simulink model "CSTFM_Mclass"  (Simulink 8.5)
settings: Solver=ode1  SolverMode=SingleTasking  StartTime=0.0  StopTime=200  FixedStep=25e-6  RelTol=1e-3
libraries: dspswit3 x1
settings Model: Creator=Administrator  LastModifiedBy=Administrator
settings DataIOCC: SignalLoggingSaveFormat=Dataset  SaveOutput=off  SaveTime=off
settings OptimizationCC: BlockReduction=off  OptimizeBlockIOStorage=off  BufferReuse=off  GlobalBufferReuse=off  ExpressionFolding=off  ExpressionDepthLimit=128  LocalBlockOutputs=off
settings DebuggingCC: UnderspecifiedInitializationDetection=Simplified  MergeDetectMultiDrivingBlocksExec=error  FcnCallInpInsideContextMsg=EnableAllAsError  StateNameClashWarn=none
settings GRTTargetCC: CombineOutputUpdateFcns=on  GRTInterface=off

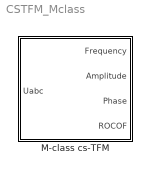
== system CSTFM_Mclass ==
  M-class cs-TFM : Subsystem  SystemSampleTime=2e-4  VariantControl=variant1  mask{nominal_freq=50, Fs=5e3, T=0.1, Fr_50=50}
      mask prompts: nominal_freq "Norminal Frequency"; Fs "Sampling rate (Hz)"; T "Window length (s)"; Fr_50 "Data report rate (frames/s)"
      mask init:
      | %% // PUM initialization//
      | % the file is used to set basic paramters and creat initial matrix  
      | % ** 2018-08-07 YIHUI ZUO
      | 
      | %% basic paramters%
      | %nominal_freq = 50;
      | %T=0.1;
      | TdF=10;
      | % data_rate_50=1; %case: 1(10),2(25),3(50)
      | %Fs=5e3;
      | P=11;
      | 
      | %% creat intial matrix
      | f0 = nominal_freq;
      | 
      | % switch data_rate_50
      | % case 1
      | % Fr_50 = 10;
      | % case 2
      | % Fr_50 = 25;
      | % case 3
      | % Fr_50 = 50;
      | % otherwise
      | % display('Non contemplated data reporting rate')
      | % end
      | 
      | Ts=1/Fs;
      | dF = 1/T;
      | M = round(T*Fs);
      | overlap=4*M/5;
      | kmax = round(f0*T);
      | k = kmax-4:kmax+12;
      | Wk = exp(-1i*2*pi*k./M);
      | NumIters=2;
      | Fr = Fr_50;
      | Tr = 1/Fr;
      | H = M*P;
      | 
      | h_axis = 0:Fs/H:Fs*(H-1)/H; % matrix h_aixs
      | 
      | D = zeros(M,H);%
      | for k = 0:M-1
      |     for h = 0:H-1
      |     esp = k - M*h/H;
      |     esp = esp*(M-1)/M;
      |     a = pi*(k-(h/H)*M);
      |     b = a/M;
      |     if b == pi || b == 0
      |         s = 1;
      |     else
      |         s = sin(a)/(M*sin(b));
      |     end
      |     D(k+1,h+1) = s*exp(-1i*pi*esp);
      |     end
      | end
      | 
      | D_funda=D(2:17,51:61);%
      | D_funda=D_funda'; 
      | inter_index=[12 17 23 28 83 89 94 100];
      | D_inter=D(2:17,inter_index);
      | D_inter=D_inter';
      | f_fund=h_axis(51:61);
      | dft_rec=zeros(11,16);
      | freq=(10:10:160);
      | 
      | for i=1:11
      |     ff0=f_fund(i);
      |     dft_rec(i,:) =(0.5*sinc((freq-ff0)*T)+0.25*sinc((freq-ff0-1/T)*T)+0.25*sinc((freq-ff0+1/T)*T))...
      |     +  (0.5*sinc((-freq+ff0)*T)+0.25*sinc((-freq+ff0-1/T)*T)+0.25*sinc((-freq+ff0+1/T)*T));
      | end
      | 
      | order = 2;
      | M=3*M/5;
      | matrix_f=zeros(M,6,11);%
      | h=1;
      | Nh=M/2;
      | freq=(45:1:55);
      | for index=1:11
      |     omega1=2*pi*freq(index)/Fs;
      |     for i=0:M-1
      |         n = i - Nh;
      |         nc = 0;
      |         facts = factorial(2:-1:0);
      |         e = exp(1j*n*h*omega1);
      |         matrix_f(i+1,nc+1:nc+2*order+2,index) = [(((n*Ts).^(order:-1:0)).*e)./facts, (((n*Ts).^(0:1:order)).*e')./fliplr(facts)];
      |     end
      | end
      | 
      | matrix_har2=zeros(M,6,11); %
      | freq=2*(45:1:55);
      | for index=1:11
      |     omega1=2*pi*freq(index)/Fs;
      |     for i=0:M-1
      |         n = i - Nh;
      |         nc = 0;
      |         facts = factorial(2:-1:0);
      |         e = exp(1j*n*h*omega1);
      |         matrix_har2(i+1,nc+1:nc+2*order+2,index) = [(((n*Ts).^(order:-1:0)).*e)./facts, (((n*Ts).^(0:1:order)).*e')./fliplr(facts)];
      |     end
      | end
      | 
      | matrix_har3=zeros(M,6,11);%
      | freq=3*(45:1:55);
      | for index=1:11
      |     omega1=2*pi*freq(index)/Fs;
      |     for i=0:M-1
      |         n = i - Nh;
      |         nc = 0;
      |         facts = factorial(2:-1:0);
      |         e = exp(1j*n*h*omega1);
      |         matrix_har3(i+1,nc+1:nc+2*order+2,index) = [(((n*Ts).^(order:-1:0)).*e)./facts, (((n*Ts).^(0:1:order)).*e')./fliplr(facts)];
      |     end
      | end
      | 
      | M = round(T*Fs);
      | clear D
      mask TypeOptions Fr_50: 10 | 25 | 50

== system CSTFM_Mclass/M-class cs-TFM ==
  Uabc : Inport
  Buffer : Buffer  N=M  V=overlap  TreatMby1Signals=One channel
  Demux : Demux  Outputs=3
  M-class cs-TFM : Subsystem  TreatAsAtomicUnit=on  SystemSampleTime=Ts*(M-overlap)
  Rate Transition : RateTransition  OutPortSampleTime=2e-4
  Terminator : Terminator
  Terminator1 : Terminator
  msdft Hanning : Subsystem  TreatAsAtomicUnit=on  SystemSampleTime=2e-4
  Frequency : Outport
  Amplitude : Outport  Port=2
  Phase : Outport  Port=3
  ROCOF : Outport  Port=4
  wires:
  Demux/3 -> Terminator1/1
  Demux/2 -> Terminator/1
  Rate Transition/1 -> Buffer/1
  msdft Hanning/1(DFT) -> M-class cs-TFM/2(A)
  M-class cs-TFM/4(RoCoF) -> ROCOF/1
  M-class cs-TFM/3(frequency) -> Frequency/1
  M-class cs-TFM/2(phase_estimated) -> Phase/1
  M-class cs-TFM/1(Amplitude) -> Amplitude/1
  Buffer/1 -> M-class cs-TFM/1(buffer_a)
  Demux/1 -> msdft Hanning/1(signal), Rate Transition/1  "Ua"
  Uabc/1 -> Demux/1

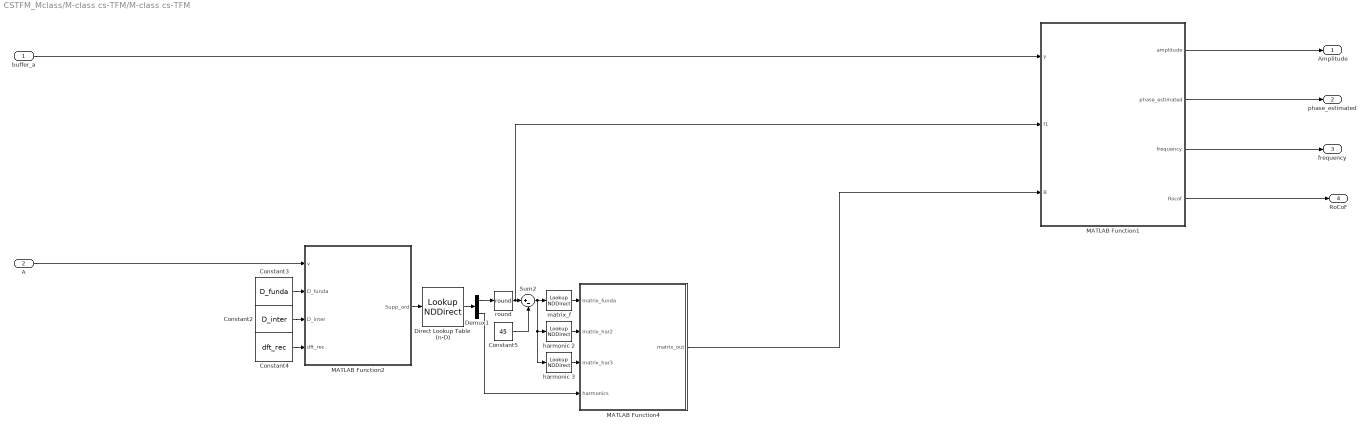
== system CSTFM_Mclass/M-class cs-TFM/M-class cs-TFM ==
  buffer_a : Inport
  A : Inport  Port=2
  Constant2 : Constant  Value=D_inter
  Constant3 : Constant  Value=D_funda
  Constant4 : Constant  Value=dft_rec
  Constant5 : Constant  Value=45
  Demux1 : Demux  Outputs=2
  Direct Lookup Table (n-D) : LookupNDDirect  NumberOfTableDimensions=1  Table=h_axis
  MATLAB Function1 : MATLAB Function  RequirementInfo={} %GIDa_19990d1e_36bc_402c_ae7c_789240e7275e  SystemSampleTime=Ts*(M-overlap)
  MATLAB Function2 : MATLAB Function  SystemSampleTime=Ts*(M-overlap)
  MATLAB Function4 : MATLAB Function  RequirementInfo={} %GIDa_4e17b5a7_f5ca_4ce2_b340_35974142e702  SystemSampleTime=Ts*(M-overlap)
  Sum2 : Sum  Inputs=|+-
  harmonic 2 : LookupNDDirect  NumberOfTableDimensions=3  InputsSelectThisObjectFromTable=2-D Matrix  Table=matrix_har2
  "harmonic 3 " : LookupNDDirect  NumberOfTableDimensions=3  InputsSelectThisObjectFromTable=2-D Matrix  Table=matrix_har3
  matrix_f : LookupNDDirect  NumberOfTableDimensions=3  InputsSelectThisObjectFromTable=2-D Matrix  Table=matrix_f
  round : Rounding  Operator=round
  Amplitude : Outport
  phase_estimated : Outport  Port=2
  frequency : Outport  Port=3
  RoCoF : Outport  Port=4
  wires:
  buffer_a/1 -> MATLAB Function1/1(y)
  round/1 -> Sum2/1, MATLAB Function1/2(f1)
  Constant3/1 -> MATLAB Function2/2(D_funda)
  MATLAB Function2/1(Supp_ord) -> Direct Lookup Table (n-D)/1
  A/1 -> MATLAB Function2/1(v)
  Constant2/1 -> MATLAB Function2/3(D_inter)
  Constant4/1 -> MATLAB Function2/4(dft_rec)
  Direct Lookup Table (n-D)/1 -> Demux1/1
  Demux1/1 -> round/1
  matrix_f/1 -> MATLAB Function4/1(matrix_funda)
  Sum2/1 -> "harmonic 3 "/1, harmonic 2/1, matrix_f/1
  Constant5/1 -> Sum2/2
  harmonic 2/1 -> MATLAB Function4/2(matrix_har2)
  "harmonic 3 "/1 -> MATLAB Function4/3(matrix_har3)
  MATLAB Function4/1(matrix_out) -> MATLAB Function1/3(B)
  Demux1/2 -> MATLAB Function4/4(harmonics)
  MATLAB Function1/1(amplitude) -> Amplitude/1
  MATLAB Function1/2(phase_estimated) -> phase_estimated/1
  MATLAB Function1/3(frequency) -> frequency/1
  MATLAB Function1/4(Rocof) -> RoCoF/1

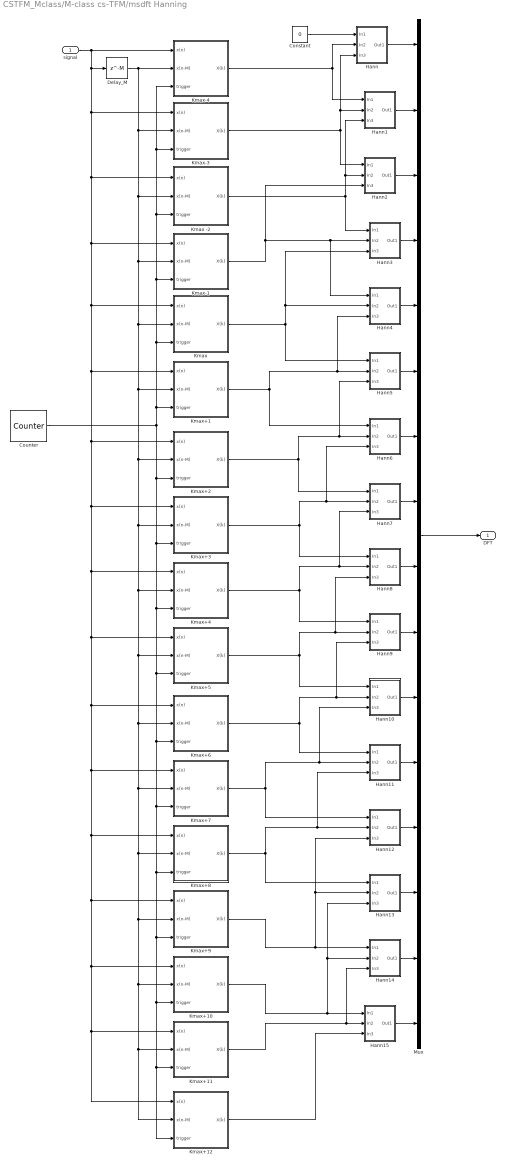
== system CSTFM_Mclass/M-class cs-TFM/msdft Hanning ==
  signal : Inport
  Constant : Constant  Value=0
  Counter : dspswit3/Counter  Direction=Up  CountEvent=Free running  CounterSize=User defined  MaxCount=M-1  InitialCount=1  Output=Hit  HitValue=0  ResetInput=off  SamplesPerFrame=1  Ts=Ts  CntDtype=double  HitDtype=Logical
  Delay_M : Delay  DelayLength=M
  Hann : Subsystem
  Hann1 : Subsystem
  Hann10 : Subsystem
  Hann11 : Subsystem
  Hann12 : Subsystem
  Hann13 : Subsystem
  Hann14 : Subsystem
  Hann15 : Subsystem
  Hann2 : Subsystem
  Hann3 : Subsystem
  Hann4 : Subsystem
  Hann5 : Subsystem
  Hann6 : Subsystem
  Hann7 : Subsystem
  Hann8 : Subsystem
  Hann9 : Subsystem
  Kmax : Subsystem
  Kmax -2 : Subsystem
  Kmax+1 : Subsystem
  Kmax+10 : Subsystem
  Kmax+11 : Subsystem
  Kmax+12 : Subsystem
  Kmax+2 : Subsystem
  Kmax+3 : Subsystem
  Kmax+4 : Subsystem
  Kmax+5 : Subsystem
  Kmax+6 : Subsystem
  Kmax+7 : Subsystem
  Kmax+8 : Subsystem
  Kmax+9 : Subsystem
  Kmax-1 : Subsystem
  Kmax-3 : Subsystem
  Kmax-4 : Subsystem
  Mux : Mux  Inputs=16
  DFT : Outport
  wires:
  Counter/1 -> Kmax+3/3(trigger), Kmax+12/3(trigger), Kmax+11/3(trigger), Kmax+10/3(trigger), Kmax+9/3(trigger), Kmax+8/3(trigger), Kmax+7/3(trigger), Kmax+6/3(trigger), Kmax+5/3(trigger), Kmax+4/3(trigger), Kmax+2/3(trigger), Kmax/3(trigger), Kmax-1/3(trigger), Kmax-3/3(trigger), Kmax-4/3(trigger), Kmax -2/3(trigger), Kmax+1/3(trigger)
  Kmax-4/1(X(k)) -> Hann/2(In2), Hann1/1(In1)
  Kmax-3/1(X(k)) -> Hann2/1(In1), Hann1/2(In2), Hann/3(In3)
  Kmax -2/1(X(k)) -> Hann3/1(In1), Hann2/2(In2), Hann1/3(In3)
  Kmax-1/1(X(k)) -> Hann2/3(In3), Hann4/1(In1), Hann3/2(In2)
  Kmax/1(X(k)) -> Hann4/2(In2), Hann3/3(In3), Hann5/1(In1)
  Kmax+2/1(X(k)) -> Hann7/1(In1), Hann5/3(In3), Hann6/2(In2)
  Kmax+4/1(X(k)) -> Hann9/1(In1), Hann7/3(In3), Hann8/2(In2)
  Kmax+11/1(X(k)) -> Hann14/3(In3), Hann15/2(In2)
  Kmax+10/1(X(k)) -> Hann13/3(In3), Hann14/2(In2), Hann15/1(In1)
  Kmax+9/1(X(k)) -> Hann12/3(In3), Hann13/2(In2), Hann14/1(In1)
  Kmax+8/1(X(k)) -> Hann13/1(In1), Hann11/3(In3), Hann12/2(In2)
  Kmax+7/1(X(k)) -> Hann12/1(In1), Hann10/3(In3), Hann11/2(In2)
  Mux/1 -> DFT/1
  signal/1 -> Kmax+12/1(x(n)), Kmax+11/1(x(n)), Kmax+10/1(x(n)), Kmax+9/1(x(n)), Kmax+8/1(x(n)), Kmax+7/1(x(n)), Kmax+6/1(x(n)), Kmax+5/1(x(n)), Kmax+4/1(x(n)), Kmax+3/1(x(n)), Kmax+2/1(x(n)), Kmax+1/1(x(n)), Kmax/1(x(n)), Kmax-1/1(x(n)), Kmax -2/1(x(n)), Kmax-3/1(x(n)), Delay_M/1, Kmax-4/1(x(n))
  Delay_M/1 -> Kmax+3/2(x(n-M)), Kmax+12/2(x(n-M)), Kmax+11/2(x(n-M)), Kmax+10/2(x(n-M)), Kmax+9/2(x(n-M)), Kmax+8/2(x(n-M)), Kmax+7/2(x(n-M)), Kmax+6/2(x(n-M)), Kmax+5/2(x(n-M)), Kmax+4/2(x(n-M)), Kmax+2/2(x(n-M)), Kmax+1/2(x(n-M)), Kmax/2(x(n-M)), Kmax-1/2(x(n-M)), Kmax -2/2(x(n-M)), Kmax-3/2(x(n-M)), Kmax-4/2(x(n-M))
  Hann/1(Out1) -> Mux/1
  Constant/1 -> Hann/1(In1)
  Hann1/1(Out1) -> Mux/2
  Hann2/1(Out1) -> Mux/3
  Hann3/1(Out1) -> Mux/4
  Hann4/1(Out1) -> Mux/5
  Hann5/1(Out1) -> Mux/6
  Hann6/1(Out1) -> Mux/7
  Hann7/1(Out1) -> Mux/8
  Hann8/1(Out1) -> Mux/9
  Hann9/1(Out1) -> Mux/10
  Hann10/1(Out1) -> Mux/11
  Hann11/1(Out1) -> Mux/12
  Hann12/1(Out1) -> Mux/13
  Hann13/1(Out1) -> Mux/14
  Hann14/1(Out1) -> Mux/15
  Hann15/1(Out1) -> Mux/16
  Kmax+12/1(X(k)) -> Hann15/3(In3)
  Kmax+6/1(X(k)) -> Hann11/1(In1), Hann9/3(In3), Hann10/2(In2)
  Kmax+5/1(X(k)) -> Hann8/3(In3), Hann9/2(In2), Hann10/1(In1)
  Kmax+3/1(X(k)) -> Hann8/1(In1), Hann6/3(In3), Hann7/2(In2)
  Kmax+1/1(X(k)) -> Hann4/3(In3), Hann5/2(In2), Hann6/1(In1)

== system CSTFM_Mclass/M-class cs-TFM/msdft Hanning/Hann ==
  In1 : Inport
  In2 : Inport  Port=2
  In3 : Inport  Port=3
  Gain : Gain  Gain=-0.25
  Gain1 : Gain  Gain=0.5
  Gain2 : Gain  Gain=-0.25
  Sum : Sum  Inputs=|+++
  Out1 : Outport
  wires:
  Sum/1 -> Out1/1
  In3/1 -> Gain2/1
  In1/1 -> Gain/1
  In2/1 -> Gain1/1
  Gain2/1 -> Sum/3
  Gain1/1 -> Sum/2
  Gain/1 -> Sum/1

== system CSTFM_Mclass/M-class cs-TFM/msdft Hanning/Hann1 ==
  In1 : Inport
  In2 : Inport  Port=2
  In3 : Inport  Port=3
  Gain : Gain  Gain=-0.25
  Gain1 : Gain  Gain=0.5
  Gain2 : Gain  Gain=-0.25
  Sum : Sum  Inputs=|+++
  Out1 : Outport
  wires:
  Sum/1 -> Out1/1
  In3/1 -> Gain2/1
  In1/1 -> Gain/1
  In2/1 -> Gain1/1
  Gain2/1 -> Sum/3
  Gain1/1 -> Sum/2
  Gain/1 -> Sum/1

== system CSTFM_Mclass/M-class cs-TFM/msdft Hanning/Hann10 ==
  In1 : Inport
  In2 : Inport  Port=2
  In3 : Inport  Port=3
  Gain : Gain  Gain=-0.25
  Gain1 : Gain  Gain=0.5
  Gain2 : Gain  Gain=-0.25
  Sum : Sum  Inputs=|+++
  Out1 : Outport
  wires:
  Sum/1 -> Out1/1
  In3/1 -> Gain2/1
  In1/1 -> Gain/1
  In2/1 -> Gain1/1
  Gain2/1 -> Sum/3
  Gain1/1 -> Sum/2
  Gain/1 -> Sum/1

== system CSTFM_Mclass/M-class cs-TFM/msdft Hanning/Hann11 ==
  In1 : Inport
  In2 : Inport  Port=2
  In3 : Inport  Port=3
  Gain : Gain  Gain=-0.25
  Gain1 : Gain  Gain=0.5
  Gain2 : Gain  Gain=-0.25
  Sum : Sum  Inputs=|+++
  Out1 : Outport
  wires:
  Sum/1 -> Out1/1
  In3/1 -> Gain2/1
  In1/1 -> Gain/1
  In2/1 -> Gain1/1
  Gain2/1 -> Sum/3
  Gain1/1 -> Sum/2
  Gain/1 -> Sum/1

== system CSTFM_Mclass/M-class cs-TFM/msdft Hanning/Hann12 ==
  In1 : Inport
  In2 : Inport  Port=2
  In3 : Inport  Port=3
  Gain : Gain  Gain=-0.25
  Gain1 : Gain  Gain=0.5
  Gain2 : Gain  Gain=-0.25
  Sum : Sum  Inputs=|+++
  Out1 : Outport
  wires:
  Sum/1 -> Out1/1
  In3/1 -> Gain2/1
  In1/1 -> Gain/1
  In2/1 -> Gain1/1
  Gain2/1 -> Sum/3
  Gain1/1 -> Sum/2
  Gain/1 -> Sum/1

== system CSTFM_Mclass/M-class cs-TFM/msdft Hanning/Hann13 ==
  In1 : Inport
  In2 : Inport  Port=2
  In3 : Inport  Port=3
  Gain : Gain  Gain=-0.25
  Gain1 : Gain  Gain=0.5
  Gain2 : Gain  Gain=-0.25
  Sum : Sum  Inputs=|+++
  Out1 : Outport
  wires:
  Sum/1 -> Out1/1
  In3/1 -> Gain2/1
  In1/1 -> Gain/1
  In2/1 -> Gain1/1
  Gain2/1 -> Sum/3
  Gain1/1 -> Sum/2
  Gain/1 -> Sum/1

== system CSTFM_Mclass/M-class cs-TFM/msdft Hanning/Hann14 ==
  In1 : Inport
  In2 : Inport  Port=2
  In3 : Inport  Port=3
  Gain : Gain  Gain=-0.25
  Gain1 : Gain  Gain=0.5
  Gain2 : Gain  Gain=-0.25
  Sum : Sum  Inputs=|+++
  Out1 : Outport
  wires:
  Sum/1 -> Out1/1
  In3/1 -> Gain2/1
  In1/1 -> Gain/1
  In2/1 -> Gain1/1
  Gain2/1 -> Sum/3
  Gain1/1 -> Sum/2
  Gain/1 -> Sum/1

== system CSTFM_Mclass/M-class cs-TFM/msdft Hanning/Hann15 ==
  In1 : Inport
  In2 : Inport  Port=2
  In3 : Inport  Port=3
  Gain : Gain  Gain=-0.25
  Gain1 : Gain  Gain=0.5
  Gain2 : Gain  Gain=-0.25
  Sum : Sum  Inputs=|+++
  Out1 : Outport
  wires:
  Sum/1 -> Out1/1
  In3/1 -> Gain2/1
  In1/1 -> Gain/1
  In2/1 -> Gain1/1
  Gain2/1 -> Sum/3
  Gain1/1 -> Sum/2
  Gain/1 -> Sum/1

== system CSTFM_Mclass/M-class cs-TFM/msdft Hanning/Hann2 ==
  In1 : Inport
  In2 : Inport  Port=2
  In3 : Inport  Port=3
  Gain : Gain  Gain=-0.25
  Gain1 : Gain  Gain=0.5
  Gain2 : Gain  Gain=-0.25
  Sum : Sum  Inputs=|+++
  Out1 : Outport
  wires:
  Sum/1 -> Out1/1
  In3/1 -> Gain2/1
  In1/1 -> Gain/1
  In2/1 -> Gain1/1
  Gain2/1 -> Sum/3
  Gain1/1 -> Sum/2
  Gain/1 -> Sum/1

== system CSTFM_Mclass/M-class cs-TFM/msdft Hanning/Hann3 ==
  In1 : Inport
  In2 : Inport  Port=2
  In3 : Inport  Port=3
  Gain : Gain  Gain=-0.25
  Gain1 : Gain  Gain=0.5
  Gain2 : Gain  Gain=-0.25
  Sum : Sum  Inputs=|+++
  Out1 : Outport
  wires:
  Sum/1 -> Out1/1
  In3/1 -> Gain2/1
  In1/1 -> Gain/1
  In2/1 -> Gain1/1
  Gain2/1 -> Sum/3
  Gain1/1 -> Sum/2
  Gain/1 -> Sum/1

== system CSTFM_Mclass/M-class cs-TFM/msdft Hanning/Hann4 ==
  In1 : Inport
  In2 : Inport  Port=2
  In3 : Inport  Port=3
  Gain : Gain  Gain=-0.25
  Gain1 : Gain  Gain=0.5
  Gain2 : Gain  Gain=-0.25
  Sum : Sum  Inputs=|+++
  Out1 : Outport
  wires:
  Sum/1 -> Out1/1
  In3/1 -> Gain2/1
  In1/1 -> Gain/1
  In2/1 -> Gain1/1
  Gain2/1 -> Sum/3
  Gain1/1 -> Sum/2
  Gain/1 -> Sum/1

== system CSTFM_Mclass/M-class cs-TFM/msdft Hanning/Hann5 ==
  In1 : Inport
  In2 : Inport  Port=2
  In3 : Inport  Port=3
  Gain : Gain  Gain=-0.25
  Gain1 : Gain  Gain=0.5
  Gain2 : Gain  Gain=-0.25
  Sum : Sum  Inputs=|+++
  Out1 : Outport
  wires:
  Sum/1 -> Out1/1
  In3/1 -> Gain2/1
  In1/1 -> Gain/1
  In2/1 -> Gain1/1
  Gain2/1 -> Sum/3
  Gain1/1 -> Sum/2
  Gain/1 -> Sum/1

== system CSTFM_Mclass/M-class cs-TFM/msdft Hanning/Hann6 ==
  In1 : Inport
  In2 : Inport  Port=2
  In3 : Inport  Port=3
  Gain : Gain  Gain=-0.25
  Gain1 : Gain  Gain=0.5
  Gain2 : Gain  Gain=-0.25
  Sum : Sum  Inputs=|+++
  Out1 : Outport
  wires:
  Sum/1 -> Out1/1
  In3/1 -> Gain2/1
  In1/1 -> Gain/1
  In2/1 -> Gain1/1
  Gain2/1 -> Sum/3
  Gain1/1 -> Sum/2
  Gain/1 -> Sum/1

== system CSTFM_Mclass/M-class cs-TFM/msdft Hanning/Hann7 ==
  In1 : Inport
  In2 : Inport  Port=2
  In3 : Inport  Port=3
  Gain : Gain  Gain=-0.25
  Gain1 : Gain  Gain=0.5
  Gain2 : Gain  Gain=-0.25
  Sum : Sum  Inputs=|+++
  Out1 : Outport
  wires:
  Sum/1 -> Out1/1
  In3/1 -> Gain2/1
  In1/1 -> Gain/1
  In2/1 -> Gain1/1
  Gain2/1 -> Sum/3
  Gain1/1 -> Sum/2
  Gain/1 -> Sum/1

== system CSTFM_Mclass/M-class cs-TFM/msdft Hanning/Hann8 ==
  In1 : Inport
  In2 : Inport  Port=2
  In3 : Inport  Port=3
  Gain : Gain  Gain=-0.25
  Gain1 : Gain  Gain=0.5
  Gain2 : Gain  Gain=-0.25
  Sum : Sum  Inputs=|+++
  Out1 : Outport
  wires:
  Sum/1 -> Out1/1
  In3/1 -> Gain2/1
  In1/1 -> Gain/1
  In2/1 -> Gain1/1
  Gain2/1 -> Sum/3
  Gain1/1 -> Sum/2
  Gain/1 -> Sum/1

== system CSTFM_Mclass/M-class cs-TFM/msdft Hanning/Hann9 ==
  In1 : Inport
  In2 : Inport  Port=2
  In3 : Inport  Port=3
  Gain : Gain  Gain=-0.25
  Gain1 : Gain  Gain=0.5
  Gain2 : Gain  Gain=-0.25
  Sum : Sum  Inputs=|+++
  Out1 : Outport
  wires:
  Sum/1 -> Out1/1
  In3/1 -> Gain2/1
  In1/1 -> Gain/1
  In2/1 -> Gain1/1
  Gain2/1 -> Sum/3
  Gain1/1 -> Sum/2
  Gain/1 -> Sum/1

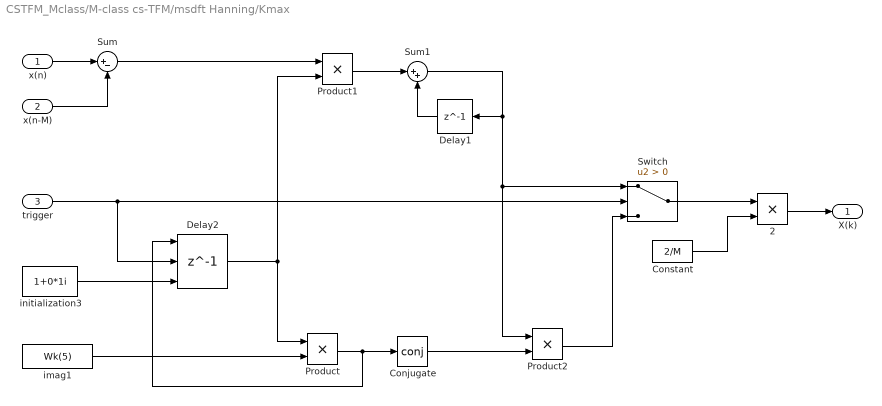
== system CSTFM_Mclass/M-class cs-TFM/msdft Hanning/Kmax ==
  x(n) : Inport
  x(n-M) : Inport  Port=2
  trigger : Inport  Port=3
  2 : Product  RndMeth=Zero
  Conjugate : Math  Operator=conj  SaturateOnIntegerOverflow=on
  Constant : Constant  Value=2/M
  Delay1 : Delay  DelayLength=1
  Delay2 : Delay  DelayLength=1  InitialConditionSource=Input port  ExternalReset=Falling
      settings: InputPortMap=u0,r5,p4
  Product : Product  RndMeth=Zero
  Product1 : Product  RndMeth=Zero
  Product2 : Product  RndMeth=Zero
  Sum : Sum  Inputs=|+-
  Sum1 : Sum  Inputs=|++
  Switch : Switch  Criteria=u2 > Threshold
  imag1 : Constant  Value=Wk(5)
  initialization3 : Constant  Value=1+0*1i
  X(k) : Outport
  wires:
  Switch/1 -> 2/1
  Product2/1 -> Switch/3
  Conjugate/1 -> Product2/2
  Product/1 -> Conjugate/1, Delay2/1
  imag1/1 -> Product/2
  initialization3/1 -> Delay2/3
  Delay2/1 -> Product/1, Product1/2
  trigger/1 -> Switch/2, Delay2/2
  2/1 -> X(k)/1
  Constant/1 -> 2/2
  Sum/1 -> Product1/1
  x(n-M)/1 -> Sum/2
  x(n)/1 -> Sum/1
  Delay1/1 -> Sum1/2
  Sum1/1 -> Product2/1, Switch/1, Delay1/1
  Product1/1 -> Sum1/1

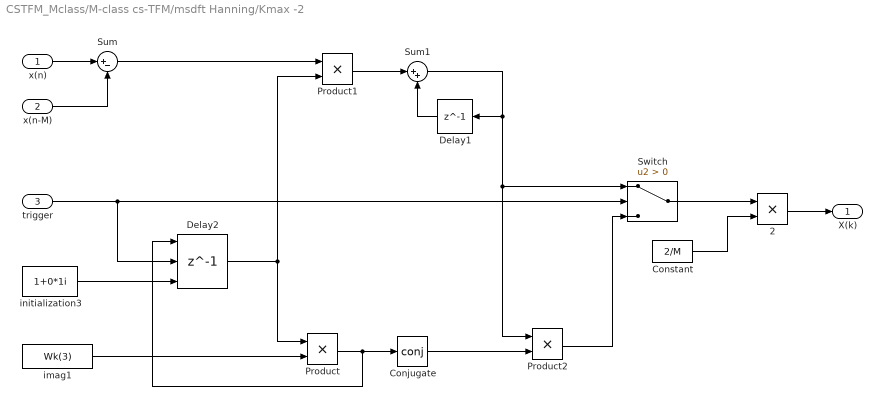
== system CSTFM_Mclass/M-class cs-TFM/msdft Hanning/Kmax -2 ==
  x(n) : Inport
  x(n-M) : Inport  Port=2
  trigger : Inport  Port=3
  2 : Product  RndMeth=Zero
  Conjugate : Math  Operator=conj  SaturateOnIntegerOverflow=on
  Constant : Constant  Value=2/M
  Delay1 : Delay  DelayLength=1
  Delay2 : Delay  DelayLength=1  InitialConditionSource=Input port  ExternalReset=Falling
      settings: InputPortMap=u0,r5,p4
  Product : Product  RndMeth=Zero
  Product1 : Product  RndMeth=Zero
  Product2 : Product  RndMeth=Zero
  Sum : Sum  Inputs=|+-
  Sum1 : Sum  Inputs=|++
  Switch : Switch  Criteria=u2 > Threshold
  imag1 : Constant  Value=Wk(3)
  initialization3 : Constant  Value=1+0*1i
  X(k) : Outport
  wires:
  Switch/1 -> 2/1
  Product2/1 -> Switch/3
  Conjugate/1 -> Product2/2
  Product/1 -> Conjugate/1, Delay2/1
  imag1/1 -> Product/2
  initialization3/1 -> Delay2/3
  Delay2/1 -> Product/1, Product1/2
  trigger/1 -> Switch/2, Delay2/2
  2/1 -> X(k)/1
  Constant/1 -> 2/2
  Sum/1 -> Product1/1
  x(n-M)/1 -> Sum/2
  x(n)/1 -> Sum/1
  Delay1/1 -> Sum1/2
  Sum1/1 -> Product2/1, Switch/1, Delay1/1
  Product1/1 -> Sum1/1

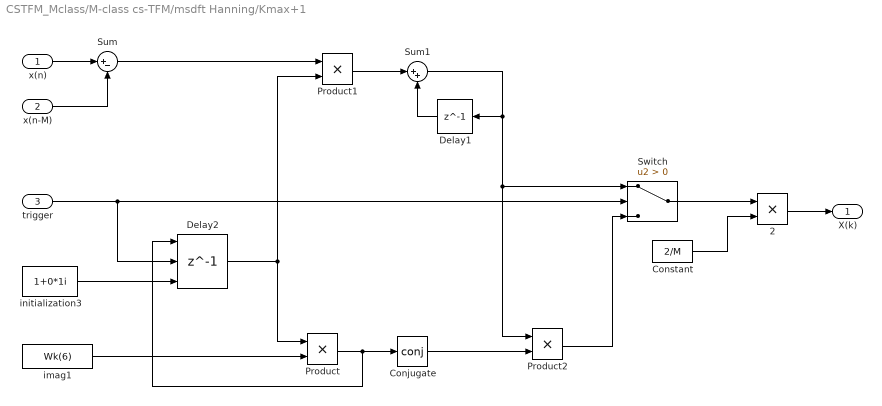
== system CSTFM_Mclass/M-class cs-TFM/msdft Hanning/Kmax+1 ==
  x(n) : Inport
  x(n-M) : Inport  Port=2
  trigger : Inport  Port=3
  2 : Product  RndMeth=Zero
  Conjugate : Math  Operator=conj  SaturateOnIntegerOverflow=on
  Constant : Constant  Value=2/M
  Delay1 : Delay  DelayLength=1
  Delay2 : Delay  DelayLength=1  InitialConditionSource=Input port  ExternalReset=Falling
      settings: InputPortMap=u0,r5,p4
  Product : Product  RndMeth=Zero
  Product1 : Product  RndMeth=Zero
  Product2 : Product  RndMeth=Zero
  Sum : Sum  Inputs=|+-
  Sum1 : Sum  Inputs=|++
  Switch : Switch  Criteria=u2 > Threshold
  imag1 : Constant  Value=Wk(6)
  initialization3 : Constant  Value=1+0*1i
  X(k) : Outport
  wires:
  Switch/1 -> 2/1
  Product2/1 -> Switch/3
  Conjugate/1 -> Product2/2
  Product/1 -> Conjugate/1, Delay2/1
  imag1/1 -> Product/2
  initialization3/1 -> Delay2/3
  Delay2/1 -> Product/1, Product1/2
  trigger/1 -> Switch/2, Delay2/2
  2/1 -> X(k)/1
  Constant/1 -> 2/2
  Sum/1 -> Product1/1
  x(n-M)/1 -> Sum/2
  x(n)/1 -> Sum/1
  Delay1/1 -> Sum1/2
  Sum1/1 -> Product2/1, Switch/1, Delay1/1
  Product1/1 -> Sum1/1

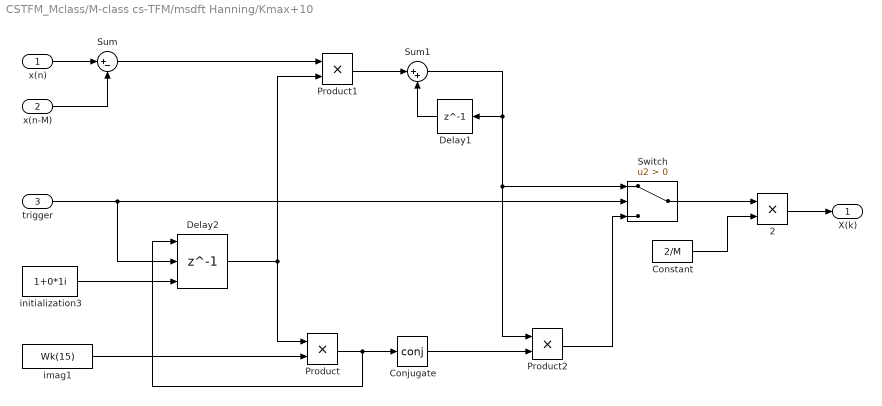
== system CSTFM_Mclass/M-class cs-TFM/msdft Hanning/Kmax+10 ==
  x(n) : Inport
  x(n-M) : Inport  Port=2
  trigger : Inport  Port=3
  2 : Product  RndMeth=Zero
  Conjugate : Math  Operator=conj  SaturateOnIntegerOverflow=on
  Constant : Constant  Value=2/M
  Delay1 : Delay  DelayLength=1
  Delay2 : Delay  DelayLength=1  InitialConditionSource=Input port  ExternalReset=Falling
      settings: InputPortMap=u0,r5,p4
  Product : Product  RndMeth=Zero
  Product1 : Product  RndMeth=Zero
  Product2 : Product  RndMeth=Zero
  Sum : Sum  Inputs=|+-
  Sum1 : Sum  Inputs=|++
  Switch : Switch  Criteria=u2 > Threshold
  imag1 : Constant  Value=Wk(15)
  initialization3 : Constant  Value=1+0*1i
  X(k) : Outport
  wires:
  Switch/1 -> 2/1
  Product2/1 -> Switch/3
  Conjugate/1 -> Product2/2
  Product/1 -> Conjugate/1, Delay2/1
  imag1/1 -> Product/2
  initialization3/1 -> Delay2/3
  Delay2/1 -> Product/1, Product1/2
  trigger/1 -> Switch/2, Delay2/2
  2/1 -> X(k)/1
  Constant/1 -> 2/2
  Sum/1 -> Product1/1
  x(n-M)/1 -> Sum/2
  x(n)/1 -> Sum/1
  Delay1/1 -> Sum1/2
  Sum1/1 -> Product2/1, Switch/1, Delay1/1
  Product1/1 -> Sum1/1

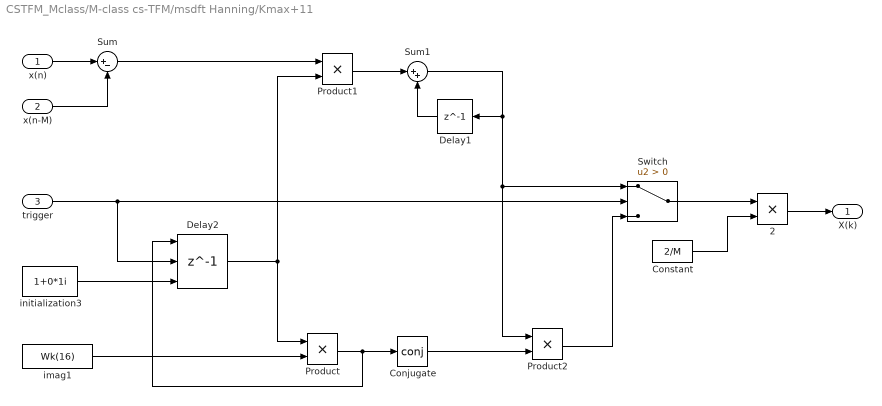
== system CSTFM_Mclass/M-class cs-TFM/msdft Hanning/Kmax+11 ==
  x(n) : Inport
  x(n-M) : Inport  Port=2
  trigger : Inport  Port=3
  2 : Product  RndMeth=Zero
  Conjugate : Math  Operator=conj  SaturateOnIntegerOverflow=on
  Constant : Constant  Value=2/M
  Delay1 : Delay  DelayLength=1
  Delay2 : Delay  DelayLength=1  InitialConditionSource=Input port  ExternalReset=Falling
      settings: InputPortMap=u0,r5,p4
  Product : Product  RndMeth=Zero
  Product1 : Product  RndMeth=Zero
  Product2 : Product  RndMeth=Zero
  Sum : Sum  Inputs=|+-
  Sum1 : Sum  Inputs=|++
  Switch : Switch  Criteria=u2 > Threshold
  imag1 : Constant  Value=Wk(16)
  initialization3 : Constant  Value=1+0*1i
  X(k) : Outport
  wires:
  Switch/1 -> 2/1
  Product2/1 -> Switch/3
  Conjugate/1 -> Product2/2
  Product/1 -> Conjugate/1, Delay2/1
  imag1/1 -> Product/2
  initialization3/1 -> Delay2/3
  Delay2/1 -> Product/1, Product1/2
  trigger/1 -> Switch/2, Delay2/2
  2/1 -> X(k)/1
  Constant/1 -> 2/2
  Sum/1 -> Product1/1
  x(n-M)/1 -> Sum/2
  x(n)/1 -> Sum/1
  Delay1/1 -> Sum1/2
  Sum1/1 -> Product2/1, Switch/1, Delay1/1
  Product1/1 -> Sum1/1

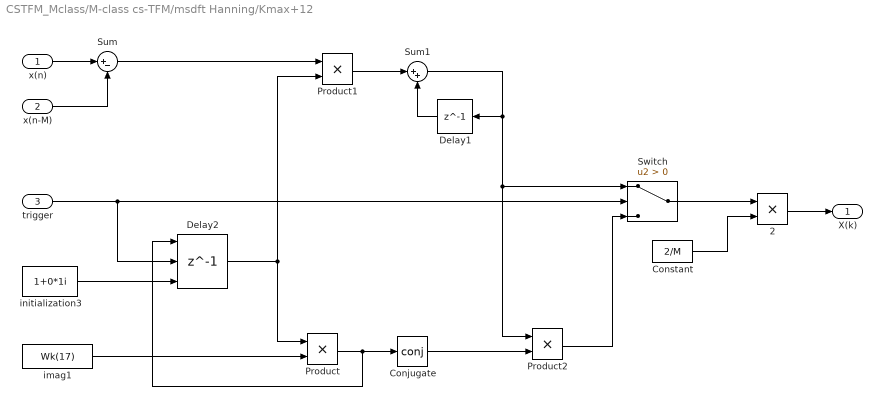
== system CSTFM_Mclass/M-class cs-TFM/msdft Hanning/Kmax+12 ==
  x(n) : Inport
  x(n-M) : Inport  Port=2
  trigger : Inport  Port=3
  2 : Product  RndMeth=Zero
  Conjugate : Math  Operator=conj  SaturateOnIntegerOverflow=on
  Constant : Constant  Value=2/M
  Delay1 : Delay  DelayLength=1
  Delay2 : Delay  DelayLength=1  InitialConditionSource=Input port  ExternalReset=Falling
      settings: InputPortMap=u0,r5,p4
  Product : Product  RndMeth=Zero
  Product1 : Product  RndMeth=Zero
  Product2 : Product  RndMeth=Zero
  Sum : Sum  Inputs=|+-
  Sum1 : Sum  Inputs=|++
  Switch : Switch  Criteria=u2 > Threshold
  imag1 : Constant  Value=Wk(17)
  initialization3 : Constant  Value=1+0*1i
  X(k) : Outport
  wires:
  Switch/1 -> 2/1
  Product2/1 -> Switch/3
  Conjugate/1 -> Product2/2
  Product/1 -> Conjugate/1, Delay2/1
  imag1/1 -> Product/2
  initialization3/1 -> Delay2/3
  Delay2/1 -> Product/1, Product1/2
  trigger/1 -> Switch/2, Delay2/2
  2/1 -> X(k)/1
  Constant/1 -> 2/2
  Sum/1 -> Product1/1
  x(n-M)/1 -> Sum/2
  x(n)/1 -> Sum/1
  Delay1/1 -> Sum1/2
  Sum1/1 -> Product2/1, Switch/1, Delay1/1
  Product1/1 -> Sum1/1

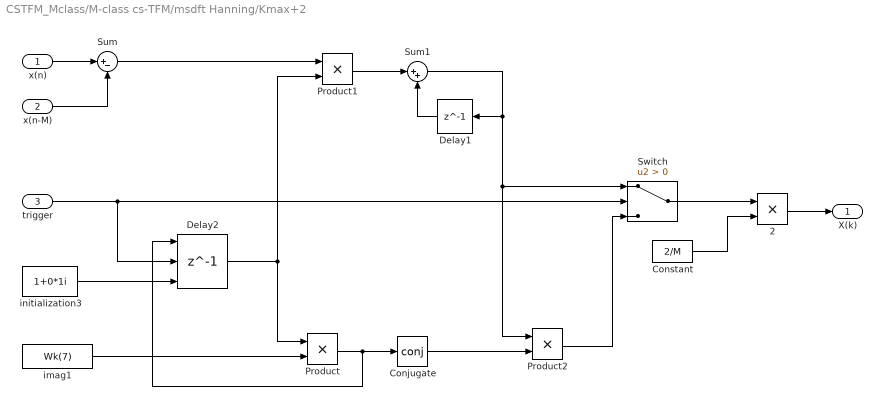
== system CSTFM_Mclass/M-class cs-TFM/msdft Hanning/Kmax+2 ==
  x(n) : Inport
  x(n-M) : Inport  Port=2
  trigger : Inport  Port=3
  2 : Product  RndMeth=Zero
  Conjugate : Math  Operator=conj  SaturateOnIntegerOverflow=on
  Constant : Constant  Value=2/M
  Delay1 : Delay  DelayLength=1
  Delay2 : Delay  DelayLength=1  InitialConditionSource=Input port  ExternalReset=Falling
      settings: InputPortMap=u0,r5,p4
  Product : Product  RndMeth=Zero
  Product1 : Product  RndMeth=Zero
  Product2 : Product  RndMeth=Zero
  Sum : Sum  Inputs=|+-
  Sum1 : Sum  Inputs=|++
  Switch : Switch  Criteria=u2 > Threshold
  imag1 : Constant  Value=Wk(7)
  initialization3 : Constant  Value=1+0*1i
  X(k) : Outport
  wires:
  Switch/1 -> 2/1
  Product2/1 -> Switch/3
  Conjugate/1 -> Product2/2
  Product/1 -> Conjugate/1, Delay2/1
  imag1/1 -> Product/2
  initialization3/1 -> Delay2/3
  Delay2/1 -> Product/1, Product1/2
  trigger/1 -> Switch/2, Delay2/2
  2/1 -> X(k)/1
  Constant/1 -> 2/2
  Sum/1 -> Product1/1
  x(n-M)/1 -> Sum/2
  x(n)/1 -> Sum/1
  Delay1/1 -> Sum1/2
  Sum1/1 -> Product2/1, Switch/1, Delay1/1
  Product1/1 -> Sum1/1

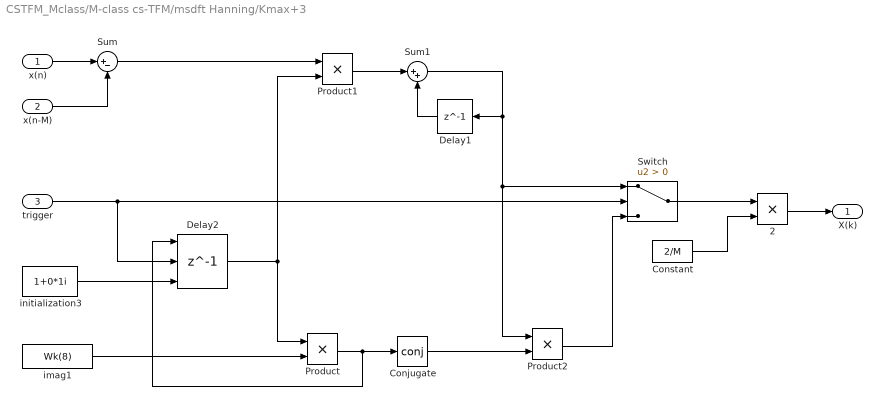
== system CSTFM_Mclass/M-class cs-TFM/msdft Hanning/Kmax+3 ==
  x(n) : Inport
  x(n-M) : Inport  Port=2
  trigger : Inport  Port=3
  2 : Product  RndMeth=Zero
  Conjugate : Math  Operator=conj  SaturateOnIntegerOverflow=on
  Constant : Constant  Value=2/M
  Delay1 : Delay  DelayLength=1
  Delay2 : Delay  DelayLength=1  InitialConditionSource=Input port  ExternalReset=Falling
      settings: InputPortMap=u0,r5,p4
  Product : Product  RndMeth=Zero
  Product1 : Product  RndMeth=Zero
  Product2 : Product  RndMeth=Zero
  Sum : Sum  Inputs=|+-
  Sum1 : Sum  Inputs=|++
  Switch : Switch  Criteria=u2 > Threshold
  imag1 : Constant  Value=Wk(8)
  initialization3 : Constant  Value=1+0*1i
  X(k) : Outport
  wires:
  Switch/1 -> 2/1
  Product2/1 -> Switch/3
  Conjugate/1 -> Product2/2
  Product/1 -> Conjugate/1, Delay2/1
  imag1/1 -> Product/2
  initialization3/1 -> Delay2/3
  Delay2/1 -> Product/1, Product1/2
  trigger/1 -> Switch/2, Delay2/2
  2/1 -> X(k)/1
  Constant/1 -> 2/2
  Sum/1 -> Product1/1
  x(n-M)/1 -> Sum/2
  x(n)/1 -> Sum/1
  Delay1/1 -> Sum1/2
  Sum1/1 -> Product2/1, Switch/1, Delay1/1
  Product1/1 -> Sum1/1

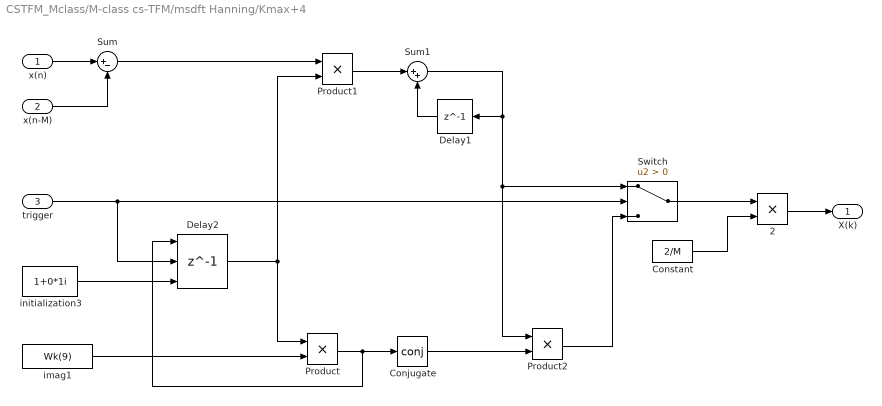
== system CSTFM_Mclass/M-class cs-TFM/msdft Hanning/Kmax+4 ==
  x(n) : Inport
  x(n-M) : Inport  Port=2
  trigger : Inport  Port=3
  2 : Product  RndMeth=Zero
  Conjugate : Math  Operator=conj  SaturateOnIntegerOverflow=on
  Constant : Constant  Value=2/M
  Delay1 : Delay  DelayLength=1
  Delay2 : Delay  DelayLength=1  InitialConditionSource=Input port  ExternalReset=Falling
      settings: InputPortMap=u0,r5,p4
  Product : Product  RndMeth=Zero
  Product1 : Product  RndMeth=Zero
  Product2 : Product  RndMeth=Zero
  Sum : Sum  Inputs=|+-
  Sum1 : Sum  Inputs=|++
  Switch : Switch  Criteria=u2 > Threshold
  imag1 : Constant  Value=Wk(9)
  initialization3 : Constant  Value=1+0*1i
  X(k) : Outport
  wires:
  Switch/1 -> 2/1
  Product2/1 -> Switch/3
  Conjugate/1 -> Product2/2
  Product/1 -> Conjugate/1, Delay2/1
  imag1/1 -> Product/2
  initialization3/1 -> Delay2/3
  Delay2/1 -> Product/1, Product1/2
  trigger/1 -> Switch/2, Delay2/2
  2/1 -> X(k)/1
  Constant/1 -> 2/2
  Sum/1 -> Product1/1
  x(n-M)/1 -> Sum/2
  x(n)/1 -> Sum/1
  Delay1/1 -> Sum1/2
  Sum1/1 -> Product2/1, Switch/1, Delay1/1
  Product1/1 -> Sum1/1

== system CSTFM_Mclass/M-class cs-TFM/msdft Hanning/Kmax+5 ==
  x(n) : Inport
  x(n-M) : Inport  Port=2
  trigger : Inport  Port=3
  2 : Product  RndMeth=Zero
  Conjugate : Math  Operator=conj  SaturateOnIntegerOverflow=on
  Constant : Constant  Value=2/M
  Delay1 : Delay  DelayLength=1
  Delay2 : Delay  DelayLength=1  InitialConditionSource=Input port  ExternalReset=Falling
      settings: InputPortMap=u0,r5,p4
  Product : Product  RndMeth=Zero
  Product1 : Product  RndMeth=Zero
  Product2 : Product  RndMeth=Zero
  Sum : Sum  Inputs=|+-
  Sum1 : Sum  Inputs=|++
  Switch : Switch  Criteria=u2 > Threshold
  imag1 : Constant  Value=Wk(10)
  initialization3 : Constant  Value=1+0*1i
  X(k) : Outport
  wires:
  Switch/1 -> 2/1
  Product2/1 -> Switch/3
  Conjugate/1 -> Product2/2
  Product/1 -> Conjugate/1, Delay2/1
  imag1/1 -> Product/2
  initialization3/1 -> Delay2/3
  Delay2/1 -> Product/1, Product1/2
  trigger/1 -> Switch/2, Delay2/2
  2/1 -> X(k)/1
  Constant/1 -> 2/2
  Sum/1 -> Product1/1
  x(n-M)/1 -> Sum/2
  x(n)/1 -> Sum/1
  Delay1/1 -> Sum1/2
  Sum1/1 -> Product2/1, Switch/1, Delay1/1
  Product1/1 -> Sum1/1

== system CSTFM_Mclass/M-class cs-TFM/msdft Hanning/Kmax+6 ==
  x(n) : Inport
  x(n-M) : Inport  Port=2
  trigger : Inport  Port=3
  2 : Product  RndMeth=Zero
  Conjugate : Math  Operator=conj  SaturateOnIntegerOverflow=on
  Constant : Constant  Value=2/M
  Delay1 : Delay  DelayLength=1
  Delay2 : Delay  DelayLength=1  InitialConditionSource=Input port  ExternalReset=Falling
      settings: InputPortMap=u0,r5,p4
  Product : Product  RndMeth=Zero
  Product1 : Product  RndMeth=Zero
  Product2 : Product  RndMeth=Zero
  Sum : Sum  Inputs=|+-
  Sum1 : Sum  Inputs=|++
  Switch : Switch  Criteria=u2 > Threshold
  imag1 : Constant  Value=Wk(11)
  initialization3 : Constant  Value=1+0*1i
  X(k) : Outport
  wires:
  Switch/1 -> 2/1
  Product2/1 -> Switch/3
  Conjugate/1 -> Product2/2
  Product/1 -> Conjugate/1, Delay2/1
  imag1/1 -> Product/2
  initialization3/1 -> Delay2/3
  Delay2/1 -> Product/1, Product1/2
  trigger/1 -> Switch/2, Delay2/2
  2/1 -> X(k)/1
  Constant/1 -> 2/2
  Sum/1 -> Product1/1
  x(n-M)/1 -> Sum/2
  x(n)/1 -> Sum/1
  Delay1/1 -> Sum1/2
  Sum1/1 -> Product2/1, Switch/1, Delay1/1
  Product1/1 -> Sum1/1

== system CSTFM_Mclass/M-class cs-TFM/msdft Hanning/Kmax+7 ==
  x(n) : Inport
  x(n-M) : Inport  Port=2
  trigger : Inport  Port=3
  2 : Product  RndMeth=Zero
  Conjugate : Math  Operator=conj  SaturateOnIntegerOverflow=on
  Constant : Constant  Value=2/M
  Delay1 : Delay  DelayLength=1
  Delay2 : Delay  DelayLength=1  InitialConditionSource=Input port  ExternalReset=Falling
      settings: InputPortMap=u0,r5,p4
  Product : Product  RndMeth=Zero
  Product1 : Product  RndMeth=Zero
  Product2 : Product  RndMeth=Zero
  Sum : Sum  Inputs=|+-
  Sum1 : Sum  Inputs=|++
  Switch : Switch  Criteria=u2 > Threshold
  imag1 : Constant  Value=Wk(12)
  initialization3 : Constant  Value=1+0*1i
  X(k) : Outport
  wires:
  Switch/1 -> 2/1
  Product2/1 -> Switch/3
  Conjugate/1 -> Product2/2
  Product/1 -> Conjugate/1, Delay2/1
  imag1/1 -> Product/2
  initialization3/1 -> Delay2/3
  Delay2/1 -> Product/1, Product1/2
  trigger/1 -> Switch/2, Delay2/2
  2/1 -> X(k)/1
  Constant/1 -> 2/2
  Sum/1 -> Product1/1
  x(n-M)/1 -> Sum/2
  x(n)/1 -> Sum/1
  Delay1/1 -> Sum1/2
  Sum1/1 -> Product2/1, Switch/1, Delay1/1
  Product1/1 -> Sum1/1

== system CSTFM_Mclass/M-class cs-TFM/msdft Hanning/Kmax+8 ==
  x(n) : Inport
  x(n-M) : Inport  Port=2
  trigger : Inport  Port=3
  2 : Product  RndMeth=Zero
  Conjugate : Math  Operator=conj  SaturateOnIntegerOverflow=on
  Constant : Constant  Value=2/M
  Delay1 : Delay  DelayLength=1
  Delay2 : Delay  DelayLength=1  InitialConditionSource=Input port  ExternalReset=Falling
      settings: InputPortMap=u0,r5,p4
  Product : Product  RndMeth=Zero
  Product1 : Product  RndMeth=Zero
  Product2 : Product  RndMeth=Zero
  Sum : Sum  Inputs=|+-
  Sum1 : Sum  Inputs=|++
  Switch : Switch  Criteria=u2 > Threshold
  imag1 : Constant  Value=Wk(13)
  initialization3 : Constant  Value=1+0*1i
  X(k) : Outport
  wires:
  Switch/1 -> 2/1
  Product2/1 -> Switch/3
  Conjugate/1 -> Product2/2
  Product/1 -> Conjugate/1, Delay2/1
  imag1/1 -> Product/2
  initialization3/1 -> Delay2/3
  Delay2/1 -> Product/1, Product1/2
  trigger/1 -> Switch/2, Delay2/2
  2/1 -> X(k)/1
  Constant/1 -> 2/2
  Sum/1 -> Product1/1
  x(n-M)/1 -> Sum/2
  x(n)/1 -> Sum/1
  Delay1/1 -> Sum1/2
  Sum1/1 -> Product2/1, Switch/1, Delay1/1
  Product1/1 -> Sum1/1

== system CSTFM_Mclass/M-class cs-TFM/msdft Hanning/Kmax+9 ==
  x(n) : Inport
  x(n-M) : Inport  Port=2
  trigger : Inport  Port=3
  2 : Product  RndMeth=Zero
  Conjugate : Math  Operator=conj  SaturateOnIntegerOverflow=on
  Constant : Constant  Value=2/M
  Delay1 : Delay  DelayLength=1
  Delay2 : Delay  DelayLength=1  InitialConditionSource=Input port  ExternalReset=Falling
      settings: InputPortMap=u0,r5,p4
  Product : Product  RndMeth=Zero
  Product1 : Product  RndMeth=Zero
  Product2 : Product  RndMeth=Zero
  Sum : Sum  Inputs=|+-
  Sum1 : Sum  Inputs=|++
  Switch : Switch  Criteria=u2 > Threshold
  imag1 : Constant  Value=Wk(14)
  initialization3 : Constant  Value=1+0*1i
  X(k) : Outport
  wires:
  Switch/1 -> 2/1
  Product2/1 -> Switch/3
  Conjugate/1 -> Product2/2
  Product/1 -> Conjugate/1, Delay2/1
  imag1/1 -> Product/2
  initialization3/1 -> Delay2/3
  Delay2/1 -> Product/1, Product1/2
  trigger/1 -> Switch/2, Delay2/2
  2/1 -> X(k)/1
  Constant/1 -> 2/2
  Sum/1 -> Product1/1
  x(n-M)/1 -> Sum/2
  x(n)/1 -> Sum/1
  Delay1/1 -> Sum1/2
  Sum1/1 -> Product2/1, Switch/1, Delay1/1
  Product1/1 -> Sum1/1

== system CSTFM_Mclass/M-class cs-TFM/msdft Hanning/Kmax-1 ==
  x(n) : Inport
  x(n-M) : Inport  Port=2
  trigger : Inport  Port=3
  2 : Product  RndMeth=Zero
  Conjugate : Math  Operator=conj  SaturateOnIntegerOverflow=on
  Constant : Constant  Value=2/M
  Delay1 : Delay  DelayLength=1
  Delay2 : Delay  DelayLength=1  InitialConditionSource=Input port  ExternalReset=Falling
      settings: InputPortMap=u0,r5,p4
  Product : Product  RndMeth=Zero
  Product1 : Product  RndMeth=Zero
  Product2 : Product  RndMeth=Zero
  Sum : Sum  Inputs=|+-
  Sum1 : Sum  Inputs=|++
  Switch : Switch  Criteria=u2 > Threshold
  imag1 : Constant  Value=Wk(4)
  initialization3 : Constant  Value=1+0*1i
  X(k) : Outport
  wires:
  Switch/1 -> 2/1
  Product2/1 -> Switch/3
  Conjugate/1 -> Product2/2
  Product/1 -> Conjugate/1, Delay2/1
  imag1/1 -> Product/2
  initialization3/1 -> Delay2/3
  Delay2/1 -> Product/1, Product1/2
  trigger/1 -> Switch/2, Delay2/2
  2/1 -> X(k)/1
  Constant/1 -> 2/2
  Sum/1 -> Product1/1
  x(n-M)/1 -> Sum/2
  x(n)/1 -> Sum/1
  Delay1/1 -> Sum1/2
  Sum1/1 -> Product2/1, Switch/1, Delay1/1
  Product1/1 -> Sum1/1

== system CSTFM_Mclass/M-class cs-TFM/msdft Hanning/Kmax-3 ==
  x(n) : Inport
  x(n-M) : Inport  Port=2
  trigger : Inport  Port=3
  2 : Product  RndMeth=Zero
  Conjugate : Math  Operator=conj  SaturateOnIntegerOverflow=on
  Constant : Constant  Value=2/M
  Delay1 : Delay  DelayLength=1
  Delay2 : Delay  DelayLength=1  InitialConditionSource=Input port  ExternalReset=Falling
      settings: InputPortMap=u0,r5,p4
  Product : Product  RndMeth=Zero
  Product1 : Product  RndMeth=Zero
  Product2 : Product  RndMeth=Zero
  Sum : Sum  Inputs=|+-
  Sum1 : Sum  Inputs=|++
  Switch : Switch  Criteria=u2 > Threshold
  imag1 : Constant  Value=Wk(2)
  initialization3 : Constant  Value=1+0*1i
  X(k) : Outport
  wires:
  Switch/1 -> 2/1
  Product2/1 -> Switch/3
  Conjugate/1 -> Product2/2
  Product/1 -> Conjugate/1, Delay2/1
  imag1/1 -> Product/2
  initialization3/1 -> Delay2/3
  Delay2/1 -> Product/1, Product1/2
  trigger/1 -> Switch/2, Delay2/2
  2/1 -> X(k)/1
  Constant/1 -> 2/2
  Sum/1 -> Product1/1
  x(n-M)/1 -> Sum/2
  x(n)/1 -> Sum/1
  Delay1/1 -> Sum1/2
  Sum1/1 -> Product2/1, Switch/1, Delay1/1
  Product1/1 -> Sum1/1

== system CSTFM_Mclass/M-class cs-TFM/msdft Hanning/Kmax-4 ==
  x(n) : Inport
  x(n-M) : Inport  Port=2
  trigger : Inport  Port=3
  2 : Product  RndMeth=Zero
  Conjugate : Math  Operator=conj  SaturateOnIntegerOverflow=on
  Constant : Constant  Value=2/M
  Delay1 : Delay  DelayLength=1
  Delay2 : Delay  DelayLength=1  InitialConditionSource=Input port  ExternalReset=Falling
      settings: InputPortMap=u0,r5,p4
  Product : Product  RndMeth=Zero
  Product1 : Product  RndMeth=Zero
  Product2 : Product  RndMeth=Zero
  Sum : Sum  Inputs=|+-
  Sum1 : Sum  Inputs=|++
  Switch : Switch  Criteria=u2 > Threshold
  imag1 : Constant  Value=Wk(1)
  initialization3 : Constant  Value=1+0*1i
  X(k) : Outport
  wires:
  Switch/1 -> 2/1
  Product2/1 -> Switch/3
  Conjugate/1 -> Product2/2
  Product/1 -> Conjugate/1, Delay2/1
  imag1/1 -> Product/2
  initialization3/1 -> Delay2/3
  Delay2/1 -> Product/1, Product1/2
  trigger/1 -> Switch/2, Delay2/2
  2/1 -> X(k)/1
  Constant/1 -> 2/2
  Sum/1 -> Product1/1
  x(n-M)/1 -> Sum/2
  x(n)/1 -> Sum/1
  Delay1/1 -> Sum1/2
  Sum1/1 -> Product2/1, Switch/1, Delay1/1
  Product1/1 -> Sum1/1

== matlab function M-class cs-TFM/M-class cs-TFM/MATLAB Function1 ==
  data: y input double; f1 input double; amplitude output double; phase_estimated output double; frequency output double; B input double; Rocof output double
function [amplitude, phase_estimated,frequency,Rocof] = CSTFM(y,f1,B)
pstima = pinv(B)*y(101:400);
ph_0 = pstima(3,:)+conj(pstima(4,:));
ph_1 = pstima(2,:)+conj(pstima(5,:));
ph_2 = pstima(1,:)+conj(pstima(6,:));

amplitude=abs(ph_0);
phase_estimated= angle(ph_0);

%% 1st order
%der_amp=2*real(ph_1*exp(-1j*phase_estimated)); % non utilizzata per il momento
der_phase=imag(ph_1*exp(-1j*phase_estimated))/amplitude;
frequency=f1+(der_phase/(2*pi));
der_amp=2*real(ph_1.*exp(-1j*phase_estimated));
%% 2nd order
der2_phase=(imag(ph_2.*exp(-1j*phase_estimated)) ...
        - 2*der_amp.*der_phase)./(amplitude); % seconda derivata fase
Rocof= der2_phase/(2*pi); % stima rocof, Hz/s
end

== matlab function M-class cs-TFM/M-class cs-TFM/MATLAB Function2 ==
  data: v input double; D_funda input double; Supp_ord output double; D_inter input double; dft_rec input double
function Supp_ord   = RunOMP_IMEKO(v,D_funda,D_inter,dft_rec)
index_tot=[23 34 45 56 83 89 94 100];
r_funda=D_funda*(v);
[maxVal, maxPos] = max(r_funda);
Supp_ord=zeros(2,1);
Supp_ord(1) = maxPos(1)+49; %% +50-1 due to look up table 0 based
v = abs(v)-abs(maxVal*transpose(dft_rec(maxPos,:)));
r_inter=D_inter*(v);
[ma_inter,ab_inter]=max(r_inter);
if abs(ma_inter)>=0.08*abs(maxVal)
    Supp_ord(2)=index_tot(ab_inter)-1; % due to the zeroth based look-up table
else
    Supp_ord(2)=0;
end
end

== matlab function M-class cs-TFM/M-class cs-TFM/MATLAB Function4 ==
  data: matrix_funda input double; matrix_har2 input double; matrix_har3 input double; matrix_out output double; harmonics input double
function matrix_out =matrixTaylorFourier_ih2(matrix_funda, matrix_har2, matrix_har3, harmonics)
% function [matrix]=matrixTaylorFourier_ih(f1, fs, N, orders, harmonics)
% in: f1 - freq di osservazione
%     fs - freq di campionamento
%     N - numero di campioni
%     orders - vettore ordini dell'espansione di Taylor delle harmonics
%     harmonics - vector of harmonic/interharmonic indexes
%     without_sampling - flag to use Ts in the matrix columns
% out: matrix matrice di TaylorFourier
fs=5e3;
if harmonics >5
    Ts=1/fs;
    numcoH =12;
    N=300;
    order=2;
    matrix = complex(zeros(N, numcoH/2));
    Nh=N/2;
    for i=0:N-1
        n = i - Nh;
        nc = 0;
        h=harmonics;
        facts = factorial(order:-1:0);
        if (h==0) % continuous component
            nc = order + 1;
            matrix(i+1,1:nc) = ((n*Ts).^(order:-1:0))./facts;
        else
            e = exp(1j*n*h*2*pi/fs);
            matrix(i+1,nc+1:nc+2*order+2) = [(((n*Ts).^(order:-1:0)).*e)./facts, (((n*Ts).^(0:1:order)).*e')./fliplr(facts)];
            nc = nc+2*order+2;
        end
    end
    matrix_out=[matrix_funda matrix_har2 matrix_har3 matrix];
else
    matrix_out=[matrix_funda matrix_har2 matrix_har3 zeros(300,6)];
end
end
